simulink model "pind1"  (Simulink 7.4)
settings: Solver=ode4  StartTime=0.0  StopTime=inf  FixedStep=0.01  RelTol=1e-3
values from neighbouring files (symbols this model uses):
  aarm = 15.836    [maaledataopsamling.m]
undefined symbols (not defined in the file or in its folder): apind
libraries: xpcnilib x1, xpclib x1
settings Model: Creator=Skov  LastModifiedBy=Skov  SimulationMode=external  BufferReuse=off
settings DataIOCC: SaveState=on  InspectSignalLogs=on
settings OptimizationCC: BlockReduction=off  OptimizeBlockIOStorage=off  BufferReuse=off  ExpressionFolding=off  LocalBlockOutputs=off
settings HardwareCC: ProdIntDivRoundTo=Zero  ProdEndianess=LittleEndian  ProdHWDeviceType=Generic->32-bit x86 compatible
settings RTWCC: SystemTargetFile=xpctarget.tlc  TemplateMakefile=xpc_default_tmf  Description=xPC Target  ProcessScript=xpctarget_make_rtw_hook  RTWCompilerOptimization=On
settings xpcTargetCC: TargetFcnLib=ansi_tfl_table_tmw.mat  TargetFunctionLibrary=ANSI_C  ParMdlRefBuildCompliant=off  PortableWordSizes=off  xPCLoadParamSetFile=off

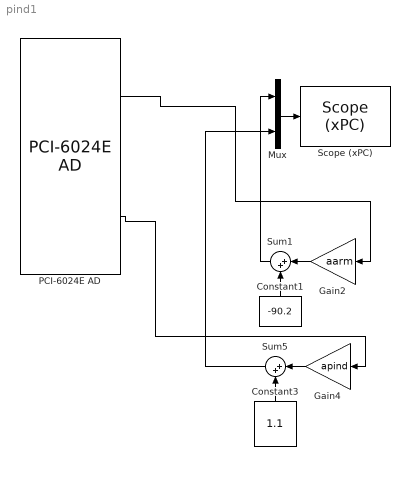
== system pind1 ==
  Constant1 : Constant  Value=-90.2  OutDataType=fixdt(1, 16)  OutScaling=2^0
  Constant3 : Constant  Value=1.1  OutDataType=fixdt(1, 16)  OutScaling=2^0
  Gain2 : Gain  Gain=aarm  ParameterDataType=fixdt(1, 16)  ParameterScaling=2^0  OutDataType=fixdt(1, 16)  OutScaling=2^0
  Gain4 : Gain  Gain=apind  ParameterDataType=fixdt(1, 16)  ParameterScaling=2^0  OutDataType=fixdt(1, 16)  OutScaling=2^0
  Mux : Mux  Inputs=2
  PCI-6024E AD : xpcnilib/A//D/E Series/PCI-6024E AD  channel=[1 2]  range=[-10]  coupling=[0]  sampletime=0.01  slot=-1
  "Scope (xPC) " : xpclib/Misc./Scope (xPC)   SystemSampleTime=-1  scopeno=1  scopetype=Target  autostart=on  viewmode=Numerical  formatstr='%15.6f'  grid=on  ylimits=[-5,5]  nosamples=250  noprepostsamples=0  interleave=1  triggermode=FreeRun  triggersignal=1  triggerlevel=0.0  triggerslope=Either  triggerscope=1  triggersample=0  filename=data.dat  mode=Lazy  writesize=512  autorestart=off  dynamicfilemode=off  maxwritefilesize=512*1024^2
  Sum1 : Sum  Inputs=|++  OutDataType=fixdt(1, 16)  OutScaling=2^0
  Sum5 : Sum  Inputs=|++  OutDataType=fixdt(1, 16)  OutScaling=2^0
  wires:
  PCI-6024E AD/1 -> Gain2/1
  PCI-6024E AD/2 -> Gain4/1
  Mux/1 -> "Scope (xPC) "/1
  Gain2/1 -> Sum1/1
  Constant1/1 -> Sum1/2
  Gain4/1 -> Sum5/1
  Constant3/1 -> Sum5/2
  Sum1/1 -> Mux/1
  Sum5/1 -> Mux/2
